simulink model "probthree"  (R2020b)
settings: Solver=VariableStepAuto  StartTime=0.0  StopTime=100  RelTol=1e-3
undefined symbols (not defined in the file): b, Kd, Ki, Kp, m
settings Model: DataDictionary=data.sldd  Creator=znome  LastModifiedBy=znome
settings SimscapeCC: SimscapeNormalizeSystem=off

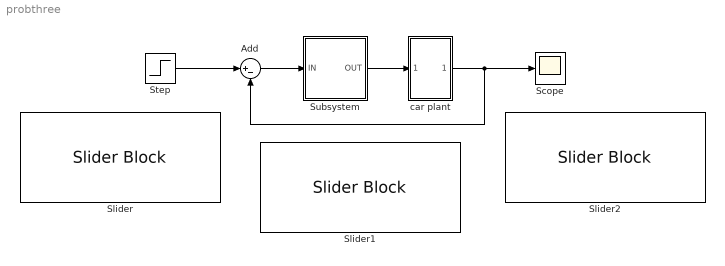
== system probthree ==
  Add : Sum  Inputs=|+-
  Scope : Scope
  Slider : SliderBlock  ScaleMin=200  ScaleMax=600
  Slider1 : SliderBlock
  Slider2 : SliderBlock  ScaleMin=500  ScaleMax=1500
  Step : Step  Time=0  After=u  SampleTime=0
  Subsystem : Subsystem  TreatAsAtomicUnit=on
  car plant : Subsystem
  wires:
  Step/1 -> Add/1
  car plant/1(Out1) -> Scope/1, Add/2
  Add/1 -> Subsystem/1(IN)
  Subsystem/1(OUT) -> car plant/1(In1)

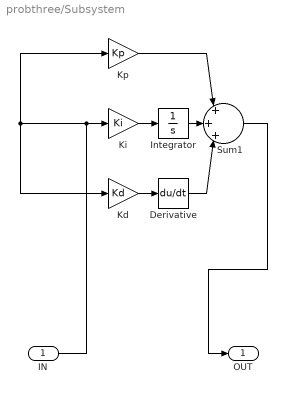
== system probthree/Subsystem ==
  IN : Inport
  Derivative : Derivative
  Integrator : Integrator
  Kd : Gain  Gain=Kd
  Ki : Gain  Gain=Ki
  Kp : Gain  Gain=Kp
  Sum1 : Sum  Inputs=|+|+|+|
  OUT : Outport
  wires:
  IN/1 -> Kp/1, Kd/1, Ki/1
  Ki/1 -> Integrator/1
  Kd/1 -> Derivative/1
  Integrator/1 -> Sum1/2
  Kp/1 -> Sum1/1
  Derivative/1 -> Sum1/3
  Sum1/1 -> OUT/1

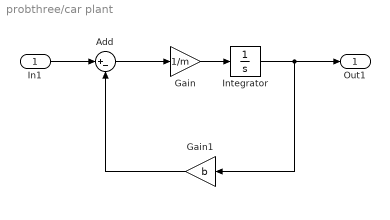
== system probthree/car plant ==
  In1 : Inport
  Add : Sum  Inputs=|+-
  Gain : Gain  Gain=1/m
  Gain1 : Gain  Gain=b
  Integrator : Integrator
  Out1 : Outport
  wires:
  Gain/1 -> Integrator/1
  Integrator/1 -> Out1/1, Gain1/1
  Gain1/1 -> Add/2
  In1/1 -> Add/1
  Add/1 -> Gain/1
